simulink model "attitude_dynamics"  (R2023a)
settings: Solver=FixedStepAuto  StartTime=0.0  StopTime=1000.0  FixedStep=0.001  RelTol=1e-3
InitFcn:
  | load('attitude_dynamics_initial.mat')
settings Model: SimulationMode=rapid-accelerator  Creator=orous  LastModifiedBy=orous
settings DataIOCC: ExternalInput=x_icrf_in,v_icrf_in,m_b_in  LoadExternalInput=on

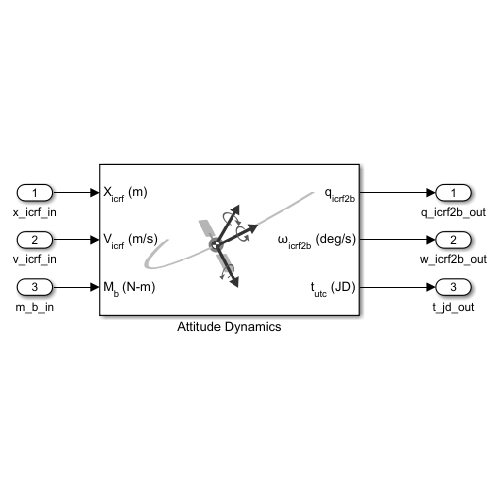
[thumbnail: Simulink's stored preview of the top-level diagram]
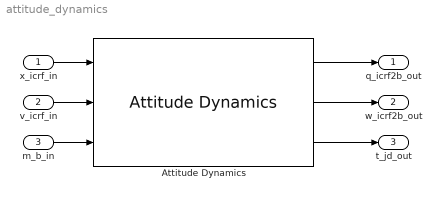
== system attitude_dynamics ==
  x_icrf_in : Inport  PortDimensions=3
  v_icrf_in : Inport  Port=2  PortDimensions=3
  m_b_in : Inport  Port=3  PortDimensions=3
  Attitude Dynamics : AttitudeDynamics
  q_icrf2b_out : Outport  PortDimensions=4
  w_icrf2b_out : Outport  Port=2  PortDimensions=3
  t_jd_out : Outport  Port=3  PortDimensions=1
  wires:
  Attitude Dynamics/1 -> q_icrf2b_out/1
  Attitude Dynamics/2 -> w_icrf2b_out/1
  v_icrf_in/1 -> Attitude Dynamics/2
  Attitude Dynamics/3 -> t_jd_out/1
  m_b_in/1 -> Attitude Dynamics/3
  x_icrf_in/1 -> Attitude Dynamics/1
